simulink model "ASDSIL"  (Simulink 7.6)
settings: Solver=FixedStepDiscrete  StartTime=0.0  StopTime=Inf  FixedStep=0.001  RelTol=1e-3
PostLoadFcn:
  | , if any(exist('dsrtsu_mdlpostloadfcn', 'file') == [2, 3, 6]), try dsrtsu_mdlpostloadfcn('Execute', bdroot); catch fprintf('Error in PostLoadFcn (dsrtsu_mdlpostloadfcn) for model "%s":\n %s\n', bdroot, lasterr); end, end,
libraries: rti1401stddiotp1cclib x2, SAEJ1939 x1, NOxSensor x1, TempSensor x1
settings Model: DSRTSU_INTERNAL_RTI_VER=370  DSRTSU_INTERNAL_RTI_TYPE=rti1401  Creator=ses  LastModifiedBy=ses  BufferReuse=off
settings OptimizationCC: BlockReduction=off  OptimizeBlockIOStorage=off  BufferReuse=off  ExpressionFolding=off  LocalBlockOutputs=off
settings HardwareCC: ProdIntDivRoundTo=Zero  ProdEndianess=BigEndian  ProdHWDeviceType=Generic->Custom  TargetIntDivRoundTo=Zero  TargetEndianess=BigEndian  TargetHWDeviceType=Generic->Custom
settings RTWCC: SystemTargetFile=rti1401.tlc  MakeCommand=make_rti  TemplateMakefile=rti1401.tmf  Description=dSPACE DS1401 Hardware Platform  ProcessScript=rti1401_make_rtw_hook
settings STFCustomTargetCC: ParMdlRefBuildCompliant=on  GeneratePreprocessorConditionals=Disable all  SystemTargetFile=rti1401.tlc
settings GRTTargetCC: CompOptLevelCompliant=off  MatFileLogging=off  ExtModeMexFile=noextcomm
settings CustomProperty: DataType=RTWOptions_EnumType_C__dSPACE_matlab_rti1401_tlc_rti1401_1InitialSimState  Value=RUN
settings EnumStrPairs: String=RUN

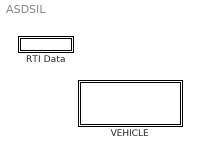
== system ASDSIL ==
  RTI Data : Subsystem  Tag=struct('RTIDataServer',struct('RTIDataServerVs','2','RTIModelDescription','struct(''main'',''ASDSIL'',''sub'','''',''isMp'',0)'))  LoadFcn="if exist('rtidc'), try,  rtidc('DataHostBlockClbLoad', gcbh); catch, disp(['Warning: ''LoadFcn'' for RTI Data block failed: ' lasterr]); end, end,"
      settings: CopyFcn="if exist('rtidc'), try,  rtidc('DataHostBlockClbCopy', gcbh); catch, disp(['Warning: ''CopyFcn'' for RTI Data block failed: ' lasterr]); end, end,"  DeleteFcn="if exist('rtidc'), try,  rtidc('DataHostBlockClbDelete', gcbh); catch, disp(['Warning: ''DeleteFcn'' for RTI Data block failed: ' lasterr]); end, end,"  ModelCloseFcn="if exist('rtidc'), try,  rtidc('DataHostBlockClbModelClose', gcbh); catch, disp(['Warning: ''ModelCloseFcn'' for RTI Data block failed: ' lasterr]); end, end,"  PreSaveFcn="if exist('rtidc'), try,  rtidc('DataHostBlockClbPreSave', gcbh); catch, disp(['Warning: ''PreSaveFcn'' for RTI Data block failed: ' lasterr]); end, end,"  PostSaveFcn="if exist('rtidc'), try,  rtidc('DataHostBlockClbPostSave', gcbh); catch, disp(['Warning: ''PostSaveFcn'' for RTI Data block failed: ' lasterr]); end, end,"  NameChangeFcn="if exist('rtidc'), try,  rtidc('DataHostBlockClbNameChange', gcbh); catch, disp(['Warning: ''NameChangeFcn'' for RTI Data block failed: ' lasterr]); end, end,"
      mask Type: RTI_DATA_HOST
      mask Description:
      | RTI Data Block.
      | This block is used by RTI to store internal model-dependent data.
      | Please keep this block on the root level of the model. Deleting this block will result in data loss.
      | 
      | NEVER DELETE OR COPY THIS BLOCK!
      mask Help:
      | RTI Data Block.
      | This block is used by RTI to store internal model-dependent data.
      | Please keep this block on the root level of the model. Deleting this block will result in data loss.
      | 
      | NEVER DELETE OR COPY THIS BLOCK!
      mask Display:
      | text(0.5, 0.5, 'RTI Data', 'HorizontalAlignment', 'center');
      | plot([1 0]);
  VEHICLE : Subsystem

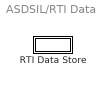
== system ASDSIL/RTI Data ==
  RTI Data Store : Subsystem  Tag="struct('private',struct('version',struct('dsVer',uint32(2),'dsVerCreation',uint32(2),'RTI',struct('ver','6.6','type','RTI1401')),'access',struct('type','Model','isPerm',1,'created',['23-Jun-2016 15:37:13'],'modified',['23-Jun-2016 16:07:11'],'location','')),'public',struct('main',struct('data',[]),'sub',struct('name',{{'ASDSIL'}},'data',{{struct('TH',struct('thTaskInfo',struct('taskType',{'TIMER','HWINT','TMRINT','SWINT'},'tasksNumOf',{2,0,0,0},'srcIds',{{'TIMERA','TIMERA2'},{},{},{}},'taskNames',{{['Timer Task 1'],['Timer Task 2']},{},{},{}})),'th_tc',struct('dataType',{'TASK','TASK'},'taskGroupId',{'',''},'taskGroupList',{{},{}},'taskSchedulingPolicy',{'FCFS','FCFS'},'taskType',{'TIMER','TIMER'},'blkh',{-1,-1},'srcId',{'TIMERA','TIMERA2'},'srcSgnName',{['Timer A interrupt'],['Timer Task 1']},'srcCpuName',{'',''},'taskName',{['Timer Task 1  [0.001] s'],['Timer Task 2  [0.1] s']},'taskNameDisplayExt',{'',''},'smplTime',{0.001,0.1},'smplTimeOffs',{0,0},'hasFixedPriority',{0,0},'priority',{1,2},'hasFixedOvc',{0,0},'ovcType',{1,1},'ovcMax',{1,1}),'tc_th',struct('dataType',{'TASK','TASK'},'taskGroupId',{'',''},'taskGroupList',{{},{}},'taskSchedulingPolicy',{'FCFS','FCFS'},'taskType',{'TIMER','TIMER'},'blkh',{-1,-1},'srcId',{'TIMERA','TIMERA2'},'srcSgnName',{['Timer A interrupt'],['Timer Task 1']},'srcCpuName',{'',''},'taskName',{['Timer Task 1  [0.001] s'],['Timer Task 2  [0.1] s']},'taskNameDisplayExt',{'',''},'smplTime',{0.001,0.1},'smplTimeOffs',{0,0},'hasFixedPriority',{0,0},'priority',{1,2},'hasFixedOvc',{0,0},'ovcType',{1,1},'ovcMax',{1,1}))}})))"
      mask Type: RTI_DATA_STORE
      mask Description:
      | RTI Data Store Block. This block is used by RTI to store internal model dependent data. Deleting this block will result in data loss.
      | 
      | NEVER DELETE, COPY, OR MODIFY THIS BLOCK!
      mask Help:
      | RTI Data Store Block. This block is used by RTI to store internal model dependent data. Deleting this block will result in data loss.
      | 
      | NEVER DELETE, COPY, OR MODIFY THIS BLOCK!
      mask Display: text(0.5, 0.5, ' ', 'HorizontalAlignment', 'center');

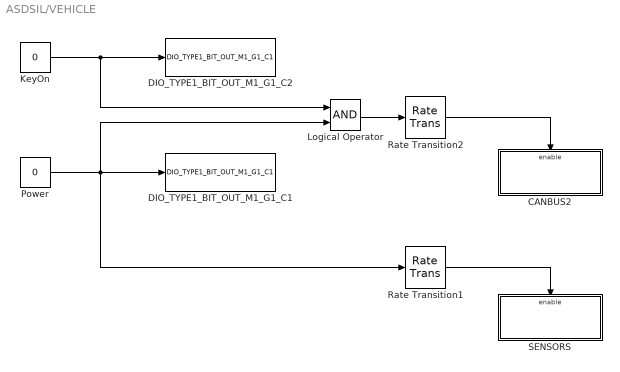
== system ASDSIL/VEHICLE ==
  CANBUS2 : Subsystem  TreatAsAtomicUnit=on
  DIO_TYPE1_BIT_OUT_M1_G1_C1 : rti1401stddiotp1cclib/DIO_TYPE1_BIT_OUT_M1_G1_C1  SystemSampleTime=-1  ModuleNo=1  BootMode=chassis ctrl  GroupNo=1  ChannelNo=1  StateInitValue=low  StateTermMode=off  StateTermValue=low  Reserved1=[]  Reserved2=[]  Reserved3=[]  Reserved4=[]  DSProperties=struct('RTI',struct('Version',uint32(5),'BlockType',struct('isSLSource',uint8(0),'isSLSink',uint8(1),'isHWSource',uint8(0),'isHWSink',uint8(1),'isSetup',uint8(0),'isInline',uint8(1),'isNonInline',uint8(1),'isInterrupt',uint8(0),'isChannelwise',uint8(1)),'IOBoardType','DS1401STANDARD','UnitType','BIT','Identifier','BITOUT','DialogType','SL','BlockSet','NONE','SlaveProcessor','MC68336'))  RTIBlockInterface=struct('InputPortsActive',1,'BlockDisplay',{{'BIT_OUT','center'}},'IconTransparency','off','InitLevel',1,'BlockName',struct('Token',{{'DIO_TYPE1_BIT_OUT_M','_G','_C'}},'BlockParam',{{'ModuleNo','GroupNo','ChannelNo'}}),'MaskDescription',['Provides bit-wise write access to the digital output.'])  RTIBlockParameters=struct('ModuleNo',{{1,'ON',[1 16]}},'BootMode',{{1,'ON',[1 5]}},'GroupNo',{{1,'ON',[1 4]}},'ChannelNo',{{1,'ON',[1 8]}},'StateInitValue',{{1,'ON',[1 2]}},'StateTermMode',{{logical(0),'ON',[0 1]}},'StateTermValue',{{1,'StateTermMode',[1 2]}})  RTISFcnParameters=struct('ModuleNo','double','BootMode','double','GroupNo','double','ChannelNo','double','StateInitValue','double','StateTermMode','double','StateTermValue','double')  RTIBlockParaDefault=struct('ModuleNo',1,'BootMode',1,'GroupNo',1,'ChannelNo',1,'StateInitValue',1,'StateTermMode',0,'StateTermValue',1)
  DIO_TYPE1_BIT_OUT_M1_G1_C2 : rti1401stddiotp1cclib/DIO_TYPE1_BIT_OUT_M1_G1_C1  SystemSampleTime=-1  ModuleNo=1  BootMode=chassis ctrl  GroupNo=1  ChannelNo=2  StateInitValue=low  StateTermMode=off  StateTermValue=low  Reserved1=[]  Reserved2=[]  Reserved3=[]  Reserved4=[]  DSProperties=struct('RTI',struct('Version',uint32(5),'BlockType',struct('isSLSource',uint8(0),'isSLSink',uint8(1),'isHWSource',uint8(0),'isHWSink',uint8(1),'isSetup',uint8(0),'isInline',uint8(1),'isNonInline',uint8(1),'isInterrupt',uint8(0),'isChannelwise',uint8(1)),'IOBoardType','DS1401STANDARD','UnitType','BIT','Identifier','BITOUT','DialogType','SL','BlockSet','NONE','SlaveProcessor','MC68336'))  RTIBlockInterface=struct('InputPortsActive',1,'BlockDisplay',{{'BIT_OUT','center'}},'IconTransparency','off','InitLevel',1,'BlockName',struct('Token',{{'DIO_TYPE1_BIT_OUT_M','_G','_C'}},'BlockParam',{{'ModuleNo','GroupNo','ChannelNo'}}),'MaskDescription',['Provides bit-wise write access to the digital output.'])  RTIBlockParameters=struct('ModuleNo',{{1,'ON',[1 16]}},'BootMode',{{1,'ON',[1 5]}},'GroupNo',{{1,'ON',[1 4]}},'ChannelNo',{{2,'ON',[1 8]}},'StateInitValue',{{1,'ON',[1 2]}},'StateTermMode',{{logical(0),'ON',[0 1]}},'StateTermValue',{{1,'StateTermMode',[1 2]}})  RTISFcnParameters=struct('ModuleNo','double','BootMode','double','GroupNo','double','ChannelNo','double','StateInitValue','double','StateTermMode','double','StateTermValue','double')  RTIBlockParaDefault=struct('ModuleNo',1,'BootMode',1,'GroupNo',1,'ChannelNo',1,'StateInitValue',1,'StateTermMode',0,'StateTermValue',1)
  KeyOn : Constant  Value=0  OutDataTypeStr=boolean
  Logical Operator : Logic  AllPortsSameDT=off  OutDataTypeStr=boolean
  Power : Constant  Value=0  OutDataTypeStr=boolean
  Rate Transition1 : RateTransition
  Rate Transition2 : RateTransition
  SENSORS : Subsystem  TreatAsAtomicUnit=on
  wires:
  Logical Operator/1 -> Rate Transition2/1
  Power/1 -> Logical Operator/2, Rate Transition1/1, DIO_TYPE1_BIT_OUT_M1_G1_C1/1
  KeyOn/1 -> Logical Operator/1, DIO_TYPE1_BIT_OUT_M1_G1_C2/1
  Rate Transition2/1 -> CANBUS2/Enable
  Rate Transition1/1 -> SENSORS/Enable

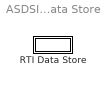
== system ASDSIL/RTI Data/RTI Data Store ==
  RTI Data Store : Subsystem
      mask Type: RTI_DATA_STORE
      mask Description:
      | RTI Data Store Block. This block is used by RTI to store internal model dependent data. Deleting this block will result in data loss.
      | 
      | NEVER DELETE, COPY, OR MODIFY THIS BLOCK!
      mask Help:
      | RTI Data Store Block. This block is used by RTI to store internal model dependent data. Deleting this block will result in data loss.
      | 
      | NEVER DELETE, COPY, OR MODIFY THIS BLOCK!
      mask Display: text(0.5, 0.5, ' ', 'HorizontalAlignment', 'center');

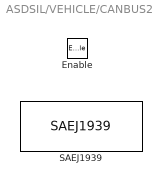
== system ASDSIL/VEHICLE/CANBUS2 ==
  Enable : EnablePort
  SAEJ1939 : SAEJ1939/SAEJ1939  SystemSampleTime=-1

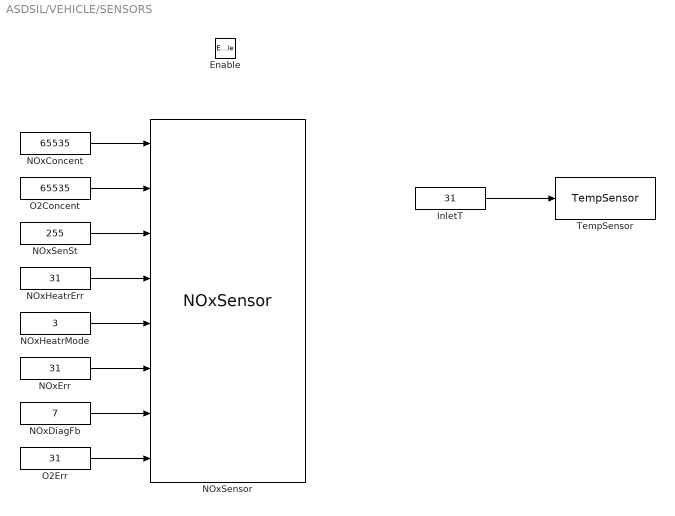
== system ASDSIL/VEHICLE/SENSORS ==
  Enable : EnablePort
  InletT : Constant  Value=31
  NOxConcent : Constant  Value=65535
  NOxDiagFb : Constant  Value=7
  NOxErr : Constant  Value=31
  NOxHeatrErr : Constant  Value=31
  NOxHeatrMode : Constant  Value=3
  NOxSenSt : Constant  Value=255
  NOxSensor : NOxSensor/NOxSensor  SystemSampleTime=-1
  O2Concent : Constant  Value=65535
  O2Err : Constant  Value=31
  TempSensor : TempSensor/TempSensor  SystemSampleTime=-1  R0=200  TSnsrVect=[1 3.8285e-3 -5.85e-7]  PuUpR=1000  PuUpU=5  CalBias=-0.006
  wires:
  NOxConcent/1 -> NOxSensor/1
  O2Concent/1 -> NOxSensor/2
  NOxSenSt/1 -> NOxSensor/3
  NOxHeatrErr/1 -> NOxSensor/4
  NOxHeatrMode/1 -> NOxSensor/5
  NOxErr/1 -> NOxSensor/6
  NOxDiagFb/1 -> NOxSensor/7
  O2Err/1 -> NOxSensor/8
  InletT/1 -> TempSensor/1

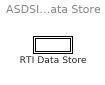
== system ASDSIL/RTI Data/RTI Data Store/RTI Data Store ==
  RTI Data Store : Subsystem
      mask Type: RTI_DATA_STORE
      mask Description:
      | RTI Data Store Block. This block is used by RTI to store internal model dependent data. Deleting this block will result in data loss.
      | 
      | NEVER DELETE, COPY, OR MODIFY THIS BLOCK!
      mask Help:
      | RTI Data Store Block. This block is used by RTI to store internal model dependent data. Deleting this block will result in data loss.
      | 
      | NEVER DELETE, COPY, OR MODIFY THIS BLOCK!
      mask Display: text(0.5, 0.5, ' ', 'HorizontalAlignment', 'center');

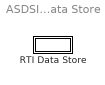
== system ASDSIL/RTI Data/RTI Data Store/RTI Data Store/RTI Data Store ==
  RTI Data Store : Subsystem
      mask Type: RTI_DATA_STORE
      mask Description:
      | RTI Data Store Block. This block is used by RTI to store internal model dependent data. Deleting this block will result in data loss.
      | 
      | NEVER DELETE, COPY, OR MODIFY THIS BLOCK!
      mask Help:
      | RTI Data Store Block. This block is used by RTI to store internal model dependent data. Deleting this block will result in data loss.
      | 
      | NEVER DELETE, COPY, OR MODIFY THIS BLOCK!
      mask Display: text(0.5, 0.5, ' ', 'HorizontalAlignment', 'center');

== system ASDSIL/RTI Data/RTI Data Store/RTI Data Store/RTI Data Store/RTI Data Store ==
